simulink model "Quadcopter_V5"  (R2024a)
settings: Solver=ode4  StartTime=0.0  StopTime=inf  FixedStep=0.01  RelTol=1e-3
undefined symbols (not defined in the file): F, MIL, Severe
libraries: slpidlib x8, simulink_extras x4, aerolibpropulsion2 x4, aerolibwind2 x2, shared6dof x1, aerolibatmos2 x1, aerolibanimutils x1, sharedtransform x1, uavutilslib x1
(part 2 of 2)

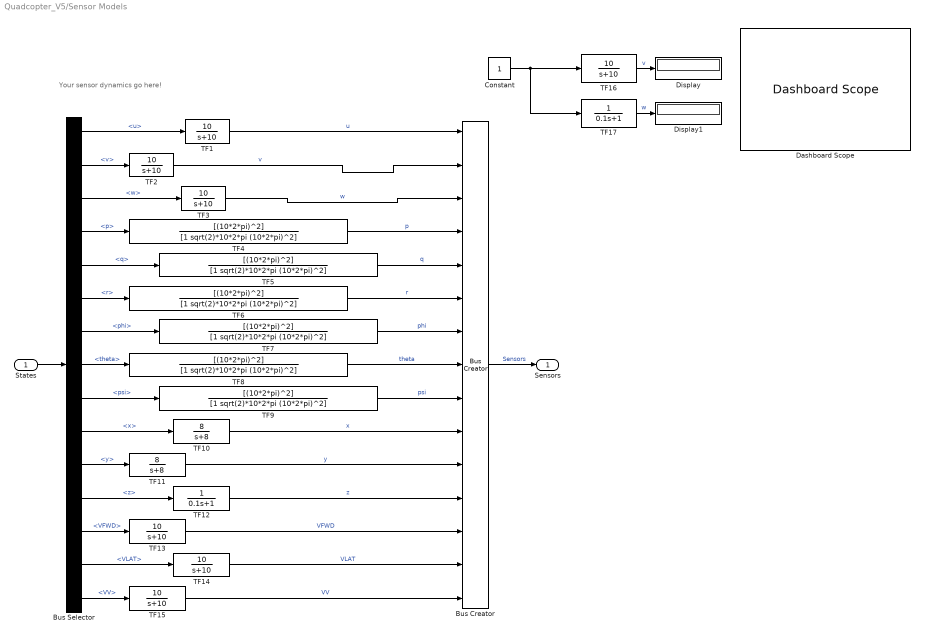
== system Quadcopter_V5/Sensor Models ==
  note: Your sensor dynamics go here!
  States : Inport
  Bus Creator : BusCreator  Inputs=15
  Bus Selector : BusSelector  OutputSignals=States.u,States.v,States.w,States.p,States.q,States.r,States.phi,States.theta,States.psi,States.x,States.y,States.z,Trajectory.VFWD,Trajectory.VLAT,Trajectory.VV
  Constant : Constant
  Dashboard Scope : DashboardScope  TimeSpan=15  Ymin=-0.1  Ymax=1.1  UpdateMode=Scroll
  Display : Display
  Display1 : Display
  TF{1..3,13..16} (7 alike) : TransferFcn  Numerator=[10]  Denominator=[1 10]
  TF10 : TransferFcn  Numerator=[8]  Denominator=[1 8]
  TF11 : TransferFcn  Numerator=[8]  Denominator=[1 8]
  TF12 : TransferFcn  Denominator=[0.1 1]
  TF17 : TransferFcn  Denominator=[0.1 1]
  TF{4..9} (6 alike) : TransferFcn  Numerator=[(10*2*pi)^2]  Denominator=[1 sqrt(2)*10*2*pi (10*2*pi)^2]
  Sensors : Outport
  wires:
  States/1 -> Bus Selector/1
  Bus Selector/1 -> TF1/1  "<u>"
  Bus Selector/2 -> TF2/1  "<v>"
  Bus Selector/3 -> TF3/1  "<w>"
  Bus Selector/4 -> TF4/1  "<p>"
  Bus Selector/5 -> TF5/1  "<q>"
  Bus Selector/6 -> TF6/1  "<r>"
  Bus Selector/7 -> TF7/1  "<phi>"
  Bus Selector/8 -> TF8/1  "<theta>"
  Bus Selector/9 -> TF9/1  "<psi>"
  Bus Selector/10 -> TF10/1  "<x>"
  Bus Selector/11 -> TF11/1  "<y>"
  Bus Selector/12 -> TF12/1  "<z>"
  TF10/1 -> Bus Creator/10  "x"
  TF1/1 -> Bus Creator/1  "u"
  TF6/1 -> Bus Creator/6  "r"
  TF2/1 -> Bus Creator/2  "v"
  TF8/1 -> Bus Creator/8  "theta"
  TF11/1 -> Bus Creator/11  "y"
  TF9/1 -> Bus Creator/9  "psi"
  TF7/1 -> Bus Creator/7  "phi"
  TF3/1 -> Bus Creator/3  "w"
  TF5/1 -> Bus Creator/5  "q"
  TF12/1 -> Bus Creator/12  "z"
  TF4/1 -> Bus Creator/4  "p"
  Bus Creator/1 -> Sensors/1  "Sensors"
  Bus Selector/13 -> TF13/1  "<VFWD>"
  TF13/1 -> Bus Creator/13  "VFWD"
  Bus Selector/14 -> TF14/1  "<VLAT>"
  TF14/1 -> Bus Creator/14  "VLAT"
  Bus Selector/15 -> TF15/1  "<VV>"
  TF15/1 -> Bus Creator/15  "VV"
  Constant/1 -> TF17/1, TF16/1
  TF16/1 -> Display/1  "v"
  TF17/1 -> Display1/1  "w"

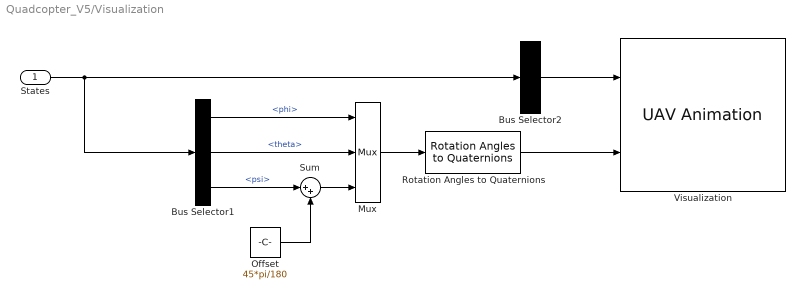
== system Quadcopter_V5/Visualization ==
  States : Inport
  Bus Selector1 : BusSelector  OutputSignals=States.phi,States.theta,States.psi
  Bus Selector2 : BusSelector  OutputSignals=States.x,States.y,States.z  OutputAsBus=on
  Mux : Mux  Inputs=3
  Offset : Constant  Value=45*pi/180
  Rotation Angles to Quaternions : sharedtransform/Rotation Angles to Quaternions  rotationOrder=XYZ  aMode=aMode
  Sum : Sum  Inputs=|++
  Visualization : uavutilslib/UAV Animation  UAVType=Multirotor  UAVSize=1  InertialZDirection=Down  SampleTime=-1
  wires:
  Rotation Angles to Quaternions/1 -> Visualization/2
  Bus Selector1/2 -> Mux/2  "<theta>"
  Bus Selector2/1 -> Visualization/1
  Bus Selector1/3 -> Sum/1  "<psi>"
  Mux/1 -> Rotation Angles to Quaternions/1
  States/1 -> Bus Selector1/1, Bus Selector2/1
  Bus Selector1/1 -> Mux/1  "<phi>"
  Sum/1 -> Mux/3
  Offset/1 -> Sum/2

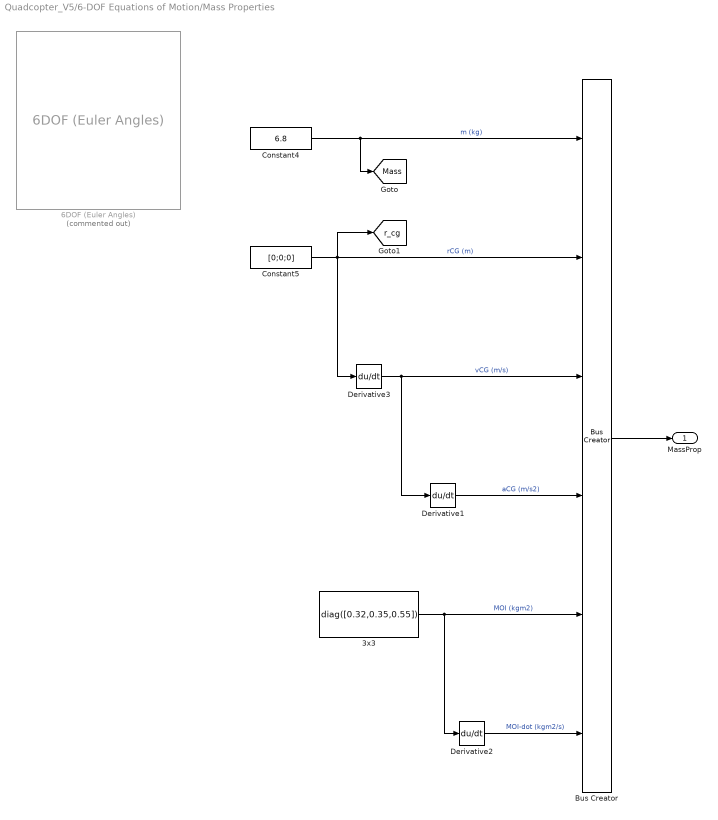
== system Quadcopter_V5/6-DOF Equations of Motion/Mass Properties ==
  3x3 : Constant  Value=diag([0.32,0.35,0.55])
  6DOF (Euler Angles) : shared6dof/6DOF (Euler Angles)  Commented=on  units=Metric (MKS)  mtype=Fixed  rep=Euler Angles  xme_0=[0 0 0]  Vm_0=[0 0 0]  eul_0=[0 0 0]  pm_0=[0 0 0]  mass_0=6.8  mass_e=0.5  mass_f=2.0  inertia=eye(3)  inertia_e=eye(3)  inertia_f=2*eye(3)  k_quat=1.0  vre_flag=on  abi_flag=off  aMode=0  xme_statename=''  Vm_statename=''  eul_statename=''  quat_statename=''  pm_statename=''  mass_statename=''
  Bus Creator : BusCreator  Inputs=6
  Constant4 : Constant  Value=6.8
  Constant5 : Constant  Value=[0;0;0]
  Derivative1 : Derivative
  Derivative2 : Derivative
  Derivative3 : Derivative
  MassProp : Outport  VectorParamsAs1DForOutWhenUnconnected=off
  tag scope: Mass=global, r_cg=global
  wires:
  Bus Creator/1 -> MassProp/1
  Constant4/1 -> [Mass], Bus Creator/1  "m (kg)"
  Derivative3/1 -> Derivative1/1, Bus Creator/3  "vCG (m/s)"
  Derivative1/1 -> Bus Creator/4  "aCG (m/s2)"
  3x3/1 -> Derivative2/1, Bus Creator/5  "MOI (kgm2)"
  Derivative2/1 -> Bus Creator/6  "MOI-dot (kgm2/s)"
  Constant5/1 -> Derivative3/1, [r_cg], Bus Creator/2  "rCG (m)"

== matlab function Quadcopter_V5/Controllers/MATLAB Function2 ==
  data: T_Cmd output; TW_Cmd input; nProps input; Weight input
function T_Cmd = fcn(TW_Cmd,nProps,Weight)

% dimensional thrust
T_Cmd = TW_Cmd*Weight/max(nProps,1);

end

== matlab function Quadcopter_V5/6-DOF Equations of Motion/EOM Integration ==
  data: X input; F_bf input; Xdot output; M_bf input; Acc output; H_bf input; H_bf_dot input; m input; MOI input; MOI_dot input; r_cg input; v_cg input; a_cg input
function [Xdot,Acc] = EOM_6DOF(X,F_bf,M_bf,H_bf,H_bf_dot,m,MOI,MOI_dot,r_cg,v_cg,a_cg)

coder.extrinsic('EOM_6DOF');
% coder.extrinsic('EOM_6DOF_OG');

Xdot = zeros(12,1);
Acc = zeros(6,1);

[Xdot,Acc,~] = EOM_6DOF(X,F_bf,M_bf,H_bf,H_bf_dot,m,MOI,MOI_dot,r_cg,v_cg,a_cg);
% [Xdot,Acc,~] = EOM_6DOF(X,F_bf,M_bf,H_bf,H_bf_dot,m,MOI,MOI_dot,r_cg,v_cg,a_cg);

end

== matlab function Quadcopter_V5/Controllers/MATLAB Function1 ==
  data: T_Cmd input; RPM output; AOI input; V_ms input; rho input; delta_RPM input
function RPM  = InverseThrustModel(T_Cmd,AOI,V_ms,rho,delta_RPM)
% inputs
% T_N: demanded thrust per propeller (N)
% V_ms: velocity normal to disk (m/s)
% rho: air density (kg/m3)
% delta_RPM: additive correction to inverse model RPM

% outputs
% RPM: predicted RPM to achieve demanded thrust

% using the angle of indicence of the flow, determine the velocity
% of the incoming flow normal to the disk (V)
% V_norm = V*cosd(AOI), where AOI is the angle of the tilting propeller
V = V_ms*cosd(AOI);

% paste the vector of coefficients here
Nvec = [1034.5       398.95       120.36      -10.519      -7.6364       11.307      0.12191      0.20162    -0.086159     -0.21103];

% % low speed fitting (1000-3000 RPM)
if T_Cmd < 2 % if requiring less than 2N of thrust, use the low speed fitting
    Nvec = [0       398.95       120.36      -10.519      -7.6364       11.307      0.12191      0.20162    -0.086159     -0.21103];
end

% execute the response surface equation
RPM_rse =   Nvec(1) +...
            Nvec(2).*T_Cmd +...
            Nvec(3).*V +...
            Nvec(4).*T_Cmd.^2 +...
            Nvec(5).*T_Cmd.*V +...
            Nvec(6).*V.^2 +...
            Nvec(7).*T_Cmd.^3 +...
            Nvec(8).*T_Cmd.^2.*V +...
            Nvec(9).*T_Cmd.*V.^2 +...
            Nvec(10).*V.^3;

% correct for air density
sigma = rho/1.225;
RPM_corr = RPM_rse/sqrt(sigma);

% add RPM correction
RPM = RPM_corr + delta_RPM;

end

== matlab function Quadcopter_V5/Force and Moment Calculations/Gravity ==
  data: m input; Fg output; phi input; theta input
function Fg = fcn(m,phi,theta)
% Gravity Model in Body Axes (3-2-1 Euler, NED convention)
%
% Inputs:
%   phi   - roll angle [rad]
%   theta - pitch angle [rad]
%
% Outputs:
%   gB    - 3x1 gravity acceleration vector in body axes [m/s^2]
%
% Notes:
%   This assumes the common aerospace convention:
%     body axes: x forward, y right, z down
%     navigation frame: NED (down positive)
%   If you need gravity *force* in body axes, use: FG = m * gB
%

% initialize outputs
Fg = zeros(3,1);

% constant gravity
g = 9.80665; % [m/s^2]

% components of gravity expressed in body axes
gx = -m * g * sin(theta);
gy =  m * g * sin(phi) * cos(theta);
gz =  m * g * cos(phi) * cos(theta);

% combine into a single output
Fg = [...
    gx;
    gy;
    gz];

end

== matlab function Quadcopter_V5/Force and Moment Calculations/Aerodynamic Drag ==
  data: S input; FD_N output; CD input; rho input; Vb input
function FD_N = fcn(S,CD,rho,Vb)
% Simple Aerodynamic Drag Model
%
% Inputs:
%   S   - reference area [m^2]
%   CD  - drag coefficient [-]
%   rho - air density [kg/m^3]
%   Vb  - body-fixed velocity vector [u; v; w] [m/s]
%
% Outputs:
%   FD         - 3x1 drag force vector in body axes [N]
%

% initialize outputs
FD_N = zeros(3,1);

% split incoming velocity vector into 3 directions:
u = Vb(1);
v = Vb(2);
w = Vb(3);

% compute drag on each axis
Fx = -1/2 * rho * S * CD * abs(u) * u;
Fy = -1/2 * rho * S * CD * abs(v) * v;
Fz = -1/2 * rho * S * CD * abs(w) * w;

% combine into a single output
FD_N = [...
    Fx;
    Fy;
    Fz];

end

== matlab function Quadcopter_V5/Force and Moment Calculations/Prop Offset Compensation ==
  data: L_Prop input; Mp_bf output; F_prop input
function Mp_bf = fcn(L_Prop,F_prop)

% initialize outputs
Mp_bf = zeros(3,1);

% grab out necessary data
Fp_bfx = F_prop(1,:)';
Fp_bfy = F_prop(2,:)';
Fp_bfz = F_prop(3,:)';

% motor hub locations (n x 1)
R = ones(4,1)*L_Prop/39.37; % R" drone arm length [m]
ps_A = [135;45;225;315]; % arm angles (from 0 --> along y axis)
x_props = R.*sind(ps_A);
y_props = R.*cosd(ps_A);
z_props = (ones(4,1) + 3)/39.37; % assume CG is below (+z) motor hubs
Prop_Loc = [x_props,y_props,z_props];

% resolve these forces into body-fixed moments (r x F expansion)
Mp_bfx = y_props.*Fp_bfz - z_props.*Fp_bfy;
Mp_bfy = z_props.*Fp_bfx - x_props.*Fp_bfz;
Mp_bfz = x_props.*Fp_bfy - y_props.*Fp_bfx;

% add across all props
Mp_x = sum(Mp_bfx);
Mp_y = sum(Mp_bfy);
Mp_z = sum(Mp_bfz);

% conactenate
Mp_bf = [...
    Mp_x;
    Mp_y;
    Mp_z];

end

== matlab function Quadcopter_V5/ESC Model/MATLAB Function ==
  data: PkW input; LoadTrq input; RPM input; I_Prop input; dRPMdt output
function dRPMdt  = MotorDynamics_MP(PkW,LoadTrq,RPM,I_Prop)

%% Initializations
nProp = 4;
Q = zeros(nProp,1);
dwdt = zeros(nProp,1);
dRPMdt = zeros(nProp,1);

% max torque
Qmax = 1.5; % Nm

%% Incoming Values
PropTorque = LoadTrq';
P_in = PkW'*1000;

% prop speed in rad/s
w = RPM*2*pi/60;

%% Standard Method
Q = P_in./w;
% limit max torque
Q = max(-Qmax,min(Q,Qmax));

% equation of motion
dwdt = (Q - PropTorque)./I_Prop;
dRPMdt = dwdt*60/(2*pi);

end

== matlab function Quadcopter_V5/Battery Model/MATLAB Function ==
  data: P_LP input; P_tot output; eta_drop input; eta output; SoC input
function [P_tot,eta] = fcn(P_LP,eta_drop,SoC)

P_tot = sum(P_LP);
PW_tot = P_tot*1000;

% with a reduction in the state of charge, the battery becomes even less efficient
SoC_factor = 1 - 0.01*(SoC - 100);
% battery efficiency is a function of total power draw and SoC
eta = 1/100*(90 - eta_drop*SoC_factor/1000*PW_tot);
% eta should never drop below a logical value
eta = max(0.3,eta);

end

== matlab function Quadcopter_V5/Controllers/MATLAB Function ==
  data: UTrimVec input; U output
function U  = ControlAllocation(UTrimVec)
%% File Information
% ControlAllocation - control allocation function (vehicle-specific)
%
% DESCRIPTION: 
%   This is a vehicle-specific control allocation (mixer) function,
%   relating normalized lateral, longitudinal, directional, and other
%   control commands to control effector commands
%
% WRITTEN BY:
%   Anthony M. Comer
%   Oklahoma State University
%   Email: anthony.m.comer@nasa.gov
%
% HISTORY:
%   07 JUL 2025 - created and debugged, AMC
%
% ***FOR INTERNAL OSU USE ONLY***
%
%% Quadplane Control Effectors

% 1. LP-1 Prop RPM
% 2. LP-2 Prop RPM
% 3. LP-3 Prop RPM
% 4. LP-4 Prop RPM

%% UTrimVec Defintion

% 1. ulat --> normalized lateral control command [-1,+1]
% 2. ulon --> normalized longitudinal control command [-1,+1]
% 3. udir --> normalized directional control command [-1,+1]
% 4. LPRPM --> common LPRPM component [0,LPRPMmax]

%% Initializations / Settings
U = zeros(4,1); % this corresponds to the number of outputs

% differential RPM limits (to be exposed)
dN_lat = 1000;
dN_lon = 1000;
dN_dir = 2500;

%% Unpack Incoming Trim Vector

ulat = UTrimVec(1);
ulon = UTrimVec(2);
udir = UTrimVec(3);
LPRPM = UTrimVec(4);

% limit possible inputs
ulat = max(-1,min(ulat,1));
ulon = max(-1,min(ulon,1));
udir = max(-1,min(udir,1));

%% Propulsor Allocation

% compute differential RPM equivalents from incoming normalized commands
dlat = ulat*dN_lat;
dlon = ulon*dN_lon;
ddir = udir*dN_dir;

% common RPM differs in forward-flight as the props shut down
LPRPM0 = LPRPM;

% propulsion mixing term
dBmat_LP = [...
    +1,+1,+1,+1;
    +1,-1,+1,-1;
    +1,+1,-1,-1;
    +1,-1,-1,+1;
    ];

% mixing matrix
% N14 = dBmat(1:4,:)*[MPRPM0;dlat*MP_roll;dlon*MP_pitch;ddir*MP_yaw];
N_LP = dBmat_LP*[LPRPM0;dlat;dlon;ddir];

% combine RPMs
N = [N_LP];

%% Form Control Effector Command Vector

U = N;

end

== matlab function Quadcopter_V5/6-DOF Equations of Motion/Output Generation ==
  data: Xdot input; X input; Accels input; States output; Velocities output; Trajectory output; Position output; AirData output; Accel output; Atmos input; h_terr input; LLA input; Angular output; LLAdot output
function [States,Velocities,Trajectory,Position,AirData,Accel,Angular,LLAdot] = Output_Model(Xdot,X,Accels,Atmos,h_terr,LLA)

States = zeros(12,1);
Velocities = zeros(6,1);
Trajectory = zeros(10,1);
Position = zeros(8,1);
AirData = zeros(4,1);
Accel = zeros(6,1);
Angular = zeros(9,1);
LLAdot = zeros(2,1);
% 
[States,Velocities,Trajectory,Position,AirData,Accel,Angular,LLAdot] = Output_Model(Xdot,X,Accels,Atmos,h_terr,LLA);

end
